simulink model "FOC1"  (R2022b)
settings: Solver=ode1  StartTime=0.0  StopTime=0.2  FixedStep=ctrlConst.TsSwitch  MaxStep=1e-6  RelTol=1e-3  EnableMultiTasking=on
undefined symbols (not defined in the file): ECM, f32_P_Coef, f32_P_Modulation, f32_P_SpdNeglimit_rpm, f32_P_SpdPoslimit_rpm, f32_P_SpeedPiMaxRatio, f32_P_SpeedPiMinRatio, FFW_enable, g_msgCore0to2_AcrKi, g_msgCore0to2_AcrKiStb, g_msgCore0to2_AcrKp, g_msgCore0to2_AcrKpStb, g_msgCore0to2_AcrSwtHiRpm, g_msgCore0to2_AcrSwtLoRpm, g_msgCore0to2_AfrKp, g_msgCore0to2_AfrTi, g_msgCore0to2_AsrKpHi, g_msgCore0to2_AsrKpLo, g_msgCore0to2_AsrSwtHiRpm, g_msgCore0to2_AsrSwtLoRpm, g_msgCore0to2_AsrTiHi, g_msgCore0to2_AsrTiLo, g_msgCore0to2_CalibEn, g_msgCore0to2_DecoupleEn, g_msgCore0to2_linearKpEn, g_msgCore0to2_maxCur, g_msgCore0to2_maxFwcCurRatio, g_msgCore0to2_maxTrq, g_msgCore0to2_pwmFrqSet, PWMFrqSwitch_C, SC_Ld_P, SC_Lq_P, SC_Psi_P, Spdratelimit_C, Tsw, u16_P_MotorPair
libraries: simulink x4, MathLib x2
(part 1 of 2)
settings Model: Creator=M00039784  LastModifiedBy=M00039784
settings SolverCC: AlgebraicLoopSolver=TrustRegion  InsertRTBMode=Never (minimum delay)
settings DataIOCC: LimitDataPoints=on  SaveFormat=Array  SaveOutput=off  SaveTime=off
settings OptimizationCC: DefaultParameterBehavior=Inlined  UseDivisionForNetSlopeComputation=on  UseFloatMulNetSlope=on  DefaultUnderspecifiedDataType=single  InlineInvariantSignals=on  PassReuseOutputArgsAs=Individual arguments  ExpressionDepthLimit=2147483647  ZeroExternalMemoryAtStartup=off  ZeroInternalMemoryAtStartup=off  NoFixptDivByZeroProtection=on  EfficientFloat2IntCast=on  LifeSpan=1  EfficientTunableParamExpr=on
settings DebuggingCC: ReadBeforeWriteMsg=DisableAll  WriteAfterWriteMsg=DisableAll  WriteAfterReadMsg=DisableAll  AlgebraicLoopMsg=none  MultiTaskDSMMsg=none  SingleTaskRateTransMsg=error  IntegerOverflowMsg=none  ParameterPrecisionLossMsg=none  FcnCallInpInsideContextMsg=warning  BusObjectLabelMismatch=none  AssertControl=DisableAll  AllowSymbolicDim=off  StateNameClashWarn=warning  SFUnexpectedBacktrackingDiag=warning  SFNoUnconditionalDefaultTransitionDiag=warning  SFExecutionAtInitializationDiag=none  SFMachineParentedDataDiag=warning  IntegerSaturationMsg=none  UnitsInconsistencyMsg=none  ArithmeticOperatorsInVariantConditions=warning
settings HardwareCC: ProdBitPerPointer=32  ProdBitPerSizeT=32  ProdBitPerPtrDiffT=32  ProdLargestAtomicFloat=None  ProdWordSize=32  ProdHWDeviceType=Infineon->TriCore
settings ModelReferenceCC: UpdateModelReferenceTargets=IfOutOfDate  EnableRefExpFcnMdlSchedulingChecks=on  ModelReferenceNumInstancesAllowed=Single  PropagateSignalLabelsOutOfModel=off
settings SFSimCC: SFSimEcho=off  SimUseLocalCustomCode=off  SimGenImportedTypeDefs=on  MATLABDynamicMemAlloc=off  CustomCodeUndefinedFunction=UseInterfaceOnly
settings RTWCC: Description=Embedded Coder  SystemTargetFile=ert.tlc  GenCodeOnly=on  GenerateMakefile=off  TemplateMakefile=ec_target.tmf  RTWVerbose=off  RTWUseLocalCustomCode=off  CodeExecutionProfiling=on  CodeProfilingSaveOptions=AllData  CodeProfilingInstrumentation=detailed
settings CodeAppCC: ForceParamTrailComments=on  IgnoreCustomStorageClasses=off  IgnoreTestpoints=on  MaxIdLength=64  SimulinkDataObjDesc=on  MATLABFcnDesc=on  CustomSymbolStrGlobalVar=pmsmfoc_rt$N$M  CustomSymbolStrType=pmsmfoc_$N$M  CustomSymbolStrFcn=$N$M$F  CustomSymbolStrFcnArg=$I$N$M  CustomSymbolStrMacro=$N$M  InsertBlockDesc=on  StateflowObjectComments=on  MATLABSourceComments=on  InternalIdentifier=Classic
settings ERTTargetCC: TargetLangStandard=C99 (ISO)  UtilityFuncGeneration=Shared location  MultiwordLength=2048  CombineSignalStateStructs=on  SupportAbsoluteTime=off  SupportNonFinite=off  SupportComplex=off  SupportNonInlinedSFcns=on  RemoveResetFunc=off  ParenthesesLevel=Maximum  GenerateASAP2=on  InlinedParameterPlacement=NonHierarchical  ERTCustomFileTemplate=example_file_process.tlc  EnableDataOwnership=on  ConvertIfToSwitch=off  SuppressUnreachableDefaultCases=off  MemSecPackage=Simulink  MemSecDataConstants=MemConst  MemSecDataParameters=MemConstVolatile
settings ConfigComp: CovMetricSettings=dcmtrzow  CovHTMLOptions=-aTS=1 -bRG=1 -bTC=1 -hTR=0 -nFC=0 -scm=1 -bcm=1 -xEv=0  CovSaveCumulativeToWorkspaceVar=on  CovSaveSingleToWorkspaceVar=on  CovExternalEMLEnable=off  CovSFcnEnable=off
settings SimscapeCC: SimscapeNormalizeSystem=off

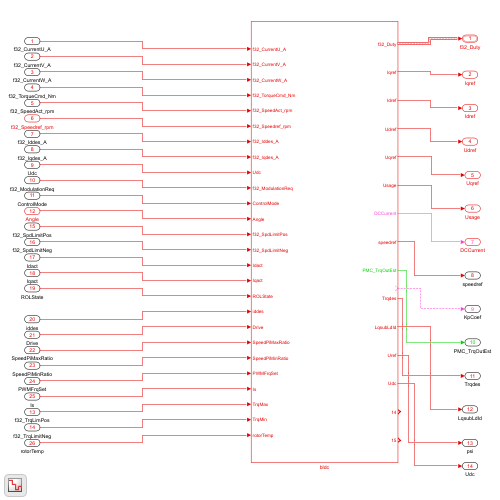
[thumbnail: Simulink's stored preview of the top-level diagram]
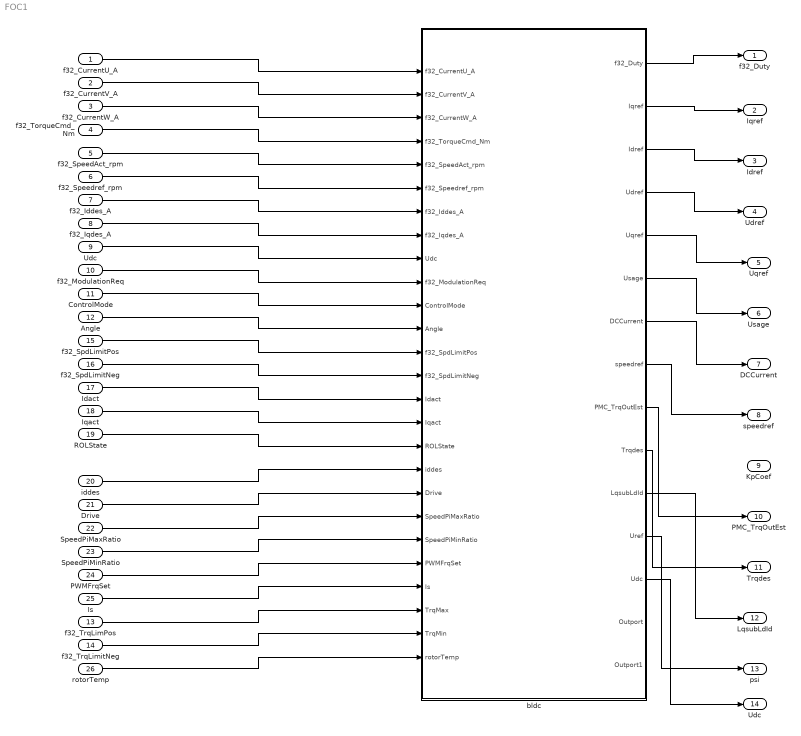
== system FOC1 ==
  f32_CurrentU_A : Inport  OutDataTypeStr=single  PortDimensions=1  SampleTime=0.0001
  f32_CurrentV_A : Inport  Port=2  OutDataTypeStr=single  PortDimensions=1  SampleTime=0.0001
  f32_CurrentW_A : Inport  Port=3  OutDataTypeStr=single  PortDimensions=1  SampleTime=0.0001
  f32_TorqueCmd_Nm : Inport  Port=4  OutDataTypeStr=single  PortDimensions=1
  f32_SpeedAct_rpm : Inport  Port=5  OutDataTypeStr=single  PortDimensions=1  SampleTime=0.0001
  f32_Speedref_rpm : Inport  Port=6  OutDataTypeStr=single  PortDimensions=1
  f32_Iddes_A : Inport  Port=7
  f32_Iqdes_A : Inport  Port=8
  "Udc " : Inport  Port=9  OutDataTypeStr=single  PortDimensions=1
  f32_ModulationReq : Inport  Port=10  OutDataTypeStr=single  PortDimensions=1
  ControlMode : Inport  Port=11  OutDataTypeStr=Enum: ECM  PortDimensions=1  SampleTime=0.0001
  Angle : Inport  Port=12  OutDataTypeStr=uint16  PortDimensions=1  SampleTime=0.0001
  f32_TrqLimPos : Inport  Port=13
  f32_TrqLimitNeg : Inport  Port=14
  f32_SpdLimitPos : Inport  Port=15
  f32_SpdLimitNeg : Inport  Port=16
  Idact : Inport  Port=17
  Iqact : Inport  Port=18
  ROLState : Inport  Port=19
  iddes : Inport  Port=20
  Drive : Inport  Port=21  OutDataTypeStr=boolean
  SpeedPiMaxRatio : Inport  Port=22  OutDataTypeStr=single
  SpeedPiMinRatio : Inport  Port=23  OutDataTypeStr=single
  PWMFrqSet : Inport  Port=24
  Is : Inport  Port=25
  rotorTemp : Inport  Port=26
  bldc : Subsystem
  f32_Duty : Outport  OutDataTypeStr=Bus: Duty
  Iqref : Outport  Port=2
  Idref : Outport  Port=3
  Udref : Outport  Port=4
  Uqref : Outport  Port=5
  Usage : Outport  Port=6
  DCCurrent : Outport  Port=7
  speedref : Outport  Port=8
  KpCoef : Outport  Port=9
  PMC_TrqOutEst : Outport  Port=10
  Trqdes : Outport  Port=11
  LqsubLdId : Outport  Port=12
  psi : Outport  Port=13
  Udc : Outport  Port=14
  wires:
  f32_SpdLimitPos/1 -> bldc/13(f32_SpdLimitPos)
  bldc/6(Usage) -> Usage/1
  f32_Speedref_rpm/1 -> bldc/6(f32_Speedref_rpm)
  f32_Iqdes_A/1 -> bldc/8(f32_Iqdes_A)
  bldc/2(Iqref) -> Iqref/1
  Angle/1 -> bldc/12(Angle)
  bldc/7(DCCurrent) -> DCCurrent/1
  bldc/5(Uqref) -> Uqref/1
  f32_SpdLimitNeg/1 -> bldc/14(f32_SpdLimitNeg)
  f32_CurrentU_A/1 -> bldc/1(f32_CurrentU_A)
  ControlMode/1 -> bldc/11(ControlMode)
  Iqact/1 -> bldc/16(Iqact)
  bldc/3(Idref) -> Idref/1
  f32_ModulationReq/1 -> bldc/10(f32_ModulationReq)
  f32_CurrentV_A/1 -> bldc/2(f32_CurrentV_A)
  bldc/1(f32_Duty) -> f32_Duty/1
  Idact/1 -> bldc/15(Idact)
  f32_TorqueCmd_Nm/1 -> bldc/4(f32_TorqueCmd_Nm)
  f32_SpeedAct_rpm/1 -> bldc/5(f32_SpeedAct_rpm)
  f32_Iddes_A/1 -> bldc/7(f32_Iddes_A)
  f32_CurrentW_A/1 -> bldc/3(f32_CurrentW_A)
  "Udc "/1 -> bldc/9("Udc ")
  bldc/4(Udref) -> Udref/1
  ROLState/1 -> bldc/17(ROLState)
  iddes/1 -> bldc/18(iddes)
  Drive/1 -> bldc/19(Drive)
  PWMFrqSet/1 -> bldc/22(PWMFrqSet)
  bldc/8(speedref) -> speedref/1
  Is/1 -> bldc/23(Is)
  ? -> KpCoef/1
  bldc/9(PMC_TrqOutEst) -> PMC_TrqOutEst/1
  f32_TrqLimPos/1 -> bldc/24(TrqMax)
  f32_TrqLimitNeg/1 -> bldc/25(TrqMin)
  SpeedPiMaxRatio/1 -> bldc/20(SpeedPiMaxRatio)
  SpeedPiMinRatio/1 -> bldc/21(SpeedPiMinRatio)
  rotorTemp/1 -> bldc/26(rotorTemp)
  bldc/10(Trqdes) -> Trqdes/1
  bldc/11(LqsubLdId) -> LqsubLdId/1
  bldc/12(Uref) -> psi/1
  bldc/13(Udc) -> Udc/1

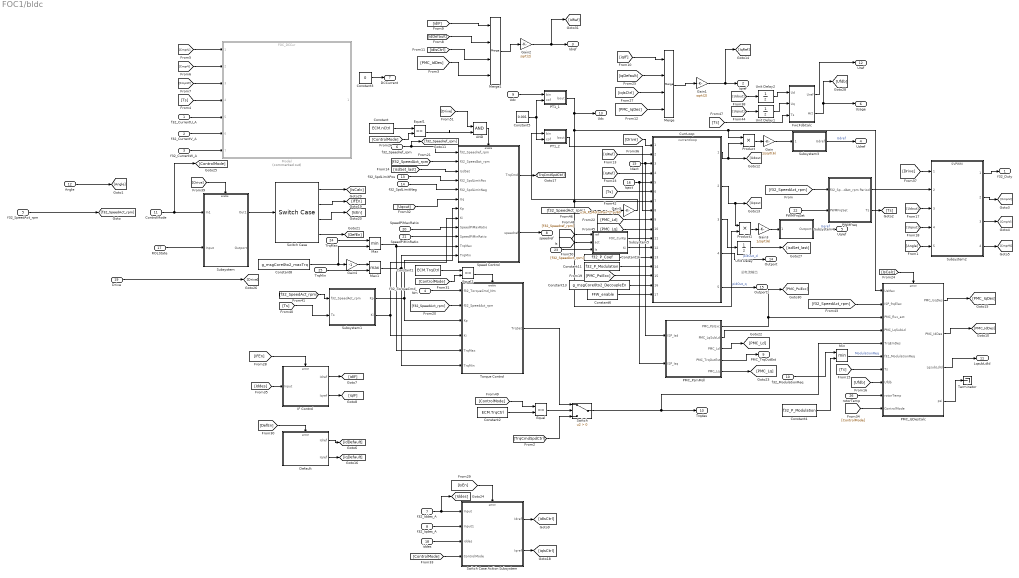
== system FOC1/bldc ==
  note: 总电流输出
  f32_CurrentU_A : Inport  OutDataTypeStr=single  PortDimensions=1  SampleTime=0.0001
  f32_CurrentV_A : Inport  Port=2  OutDataTypeStr=single  PortDimensions=1  SampleTime=0.0001
  f32_CurrentW_A : Inport  Port=3  OutDataTypeStr=single  PortDimensions=1  SampleTime=0.0001
  f32_TorqueCmd_Nm : Inport  Port=4  OutDataTypeStr=single  PortDimensions=1
  f32_SpeedAct_rpm : Inport  Port=5  OutDataTypeStr=single  PortDimensions=1  SampleTime=0.0001
  f32_Speedref_rpm : Inport  Port=6  OutDataTypeStr=single  PortDimensions=1  SampleTime=0.0001
  f32_Iddes_A : Inport  Port=7
  f32_Iqdes_A : Inport  Port=8
  "Udc " : Inport  Port=9  OutDataTypeStr=single  PortDimensions=1
  f32_ModulationReq : Inport  Port=10
  ControlMode : Inport  Port=11  OutDataTypeStr=Enum: ECM  PortDimensions=1  SampleTime=0.0001
  Angle : Inport  Port=12  OutDataTypeStr=uint16  PortDimensions=1  SampleTime=0.0001
  f32_SpdLimitPos : Inport  Port=13
  f32_SpdLimitNeg : Inport  Port=14
  Idact : Inport  Port=15
  Iqact : Inport  Port=16
  ROLState : Inport  Port=17
  iddes : Inport  Port=18
  Drive : Inport  Port=19
  SpeedPiMaxRatio : Inport  Port=20
  SpeedPiMinRatio : Inport  Port=21
  PWMFrqSet : Inport  Port=22
  Is : Inport  Port=23
  TrqMax : Inport  Port=24
  TrqMin : Inport  Port=25
  rotorTemp : Inport  Port=26
  AND : Logic  IconShape=distinctive  AllPortsSameDT=off  OutDataTypeStr=boolean
  Constant : Constant  Value=ECM.nCtrl
  Constant1 : Constant  Value=ECM.TrqCtrl
  Constant11 : Constant  Value=f32_P_Modulation
  Constant13 : Constant  Value=g_msgCore0to2_DecoupleEn
  Constant16 : Constant  Value=f32_P_Coef
  Constant2 : Constant  Value=ECM.TrqCtrl
  Constant3 : Constant  Value=0  OutDataTypeStr=single
  Constant4 : Constant  Value=f32_P_Modulation  OutDataTypeStr=single
  Constant5 : Constant  Value=0.001  OutDataTypeStr=single
  Constant6 : Constant  Value=FFW_enable
  Constant8 : Constant  Value=g_msgCore0to2_maxTrq  OutDataTypeStr=single  SampleTime=-1
  CurrLoop : ModelReference  ModelNameDialog=currentloop.slxp  ModelReferenceVersion=1.125  CopyOfModelProtected=on
  Default : Subsystem  TreatAsAtomicUnit=on
  Equal : RelationalOperator  Operator===  OutDataTypeStr=boolean  RndMeth=Simplest  InputSameDT=off
  Equal1 : RelationalOperator  Operator===  OutDataTypeStr=boolean  RndMeth=Simplest  InputSameDT=off
  Equal2 : RelationalOperator  Operator===  OutDataTypeStr=boolean  RndMeth=Simplest  InputSameDT=off
  FwcFdbCalc : Subsystem
  Gain : Gain  Gain=1/sqrt(6)
  Gain1 : Gain  Gain=sqrt(2)
  Gain2 : Gain  Gain=sqrt(2)
  Gain3 : Gain  Gain=1/sqrt(6)
  Gain4 : Gain  Gain=-1
  Gain5 : Gain  Gain=u16_P_MotorPair*2*pi/60
  IF Control : Subsystem  TreatAsAtomicUnit=on
  Max : MinMax  Inputs=2
  Max1 : MinMax  Function=max  Inputs=2
  Merge : Merge  Inputs=4  InitialOutput=0
  Merge1 : Merge  Inputs=4  InitialOutput=0
  Min : MinMax  Inputs=2
  Model : ModelReference  Commented=on  ModelNameDialog=FOC_DCCur.slx  SimulationMode=Normal  ModelReferenceVersion=1.20
  PMC_IsDesCalc : Subsystem
  PMC_PsmMdl : Subsystem
  PT1_1 : Subsystem
  PT1_2 : Subsystem
  PWMfreq : Subsystem
  Product : Product
  Product1 : Product
  Speed Control : Subsystem
  Subsystem : Subsystem
  Subsystem1 : Subsystem
  Subsystem2 : ModelReference  ModelNameDialog=SVPWM.slxp  ModelReferenceVersion=1.113  CopyOfModelProtected=on
  Subsystem3 : Subsystem
  Subsystem4 : Subsystem
  Subsystem5 : Subsystem
  Switch : Switch  Criteria=u2 > Threshold  SaturateOnIntegerOverflow=off  InputSameDT=off
  Switch Case : SwitchCase  CaseConditions={[ECM.nCtrl,ECM.TrqCtrl],ECM.IFCtrl,[ECM.IsCtrl,ECM.alOfsCal]}
  Switch Case Action Subsystem : Subsystem  TreatAsAtomicUnit=on
  Terminator : Terminator
  Torque Control : Subsystem
  Unit Delay : UnitDelay  SampleTime=-1  HasFrameUpgradeWarning=on
  Unit Delay1 : UnitDelay  SampleTime=-1  HasFrameUpgradeWarning=on
  Unit Delay2 : UnitDelay  SampleTime=-1  HasFrameUpgradeWarning=on
  f32_Duty : Outport  OutDataTypeStr=Bus: Duty
  Iqref : Outport  Port=2
  Idref : Outport  Port=3
  Udref : Outport  Port=4
  Uqref : Outport  Port=5
  Usage : Outport  Port=6
  DCCurrent : Outport  Port=7
  speedref : Outport  Port=8
  PMC_TrqOutEst : Outport  Port=9
  Trqdes : Outport  Port=10
  LqsubLdId : Outport  Port=11
  Uref : Outport  Port=12
  Udc : Outport  Port=13
  Outport : Outport  Port=14
  Outport1 : Outport  Port=15
  wires:
  Subsystem2/1 -> f32_Duty/1
  PWMfreq/1(Period) -> Subsystem2/2
  f32_CurrentW_A/1 -> Model/7
  CurrLoop/1 -> Product/2, [Udout]
  [Angle] -> Subsystem2/5
  f32_CurrentU_A/1 -> Model/5
  f32_SpeedAct_rpm/1 -> [f32_SpeedAct_rpm]
  f32_SpdLimitPos/1 -> Speed Control/4(f32_SpdLimitPos)
  f32_CurrentV_A/1 -> Model/6
  f32_SpdLimitNeg/1 -> Speed Control/5(f32_SpdLimitNeg)
  f32_Speedref_rpm/1 -> Speed Control/1(f32_Speedref_rpm), [f32_Speedref_rpm]
  CurrLoop/2 -> [Uqout], Product1/1
  PWMfreq/2(Ts) -> [Ts]
  [f32_SpeedAct_rpm] -> PWMfreq/1(f32_SpeedAct_rpm)
  ControlMode/1 -> [ControlMode], Subsystem/1(In1)
  Angle/1 -> [Angle]
  Idact/1 -> PMC_PsmMdl/1(ISP_Isd), CurrLoop/3
  Iqact/1 -> PMC_PsmMdl/2(ISP_Isq), CurrLoop/5
  [Ts] -> Model/4
  Subsystem2/2 -> [CmprU]
  Subsystem2/3 -> [CmprV]
  Subsystem2/4 -> [CmprW]
  [CmprW] -> Model/3
  [CmprV] -> Model/2
  [CmprU] -> Model/1
  Constant3/1 -> DCCurrent/1
  f32_Iddes_A/1 -> [Iddes], Switch Case Action Subsystem/1(Input)
  f32_Iqdes_A/1 -> Switch Case Action Subsystem/2(Input1)
  Default/1("Idref ") -> [idDefault]
  [idDefault] -> Merge1/2
  IF Control/1(Idref) -> [idIF]
  [idIF] -> Merge1/1
  IF Control/2(Iqref) -> [iqIF]
  Switch Case Action Subsystem/1("Idref ") -> [idIsCtrl]
  [idIsCtrl] -> Merge1/3
  [isdSet_last] -> Speed Control/3(IsdSet)
  [Udout] -> Subsystem2/3
  [Uqout] -> Subsystem2/4
  [f32_SpeedAct_rpm] -> Torque Control/2(f32_SpeedAct_rpm)
  [f32_SpeedAct_rpm] -> Speed Control/2(f32_SpeedAct_rpm)
  Merge/1 -> Gain1/1
  [IqRef] -> CurrLoop/4
  Default/2(Iqref) -> [iqDefault]
  Speed Control/1("TrqCmd ") -> [TrqCmdSpdCtrl]
  Switch Case Action Subsystem/2(Iqref) -> [iqIsCtrl]
  [IFEn] -> IF Control/Action
  Switch Case/2 -> [IFEn]
  [IsEn] -> Switch Case Action Subsystem/Action
  Switch Case/3 -> [IsEn]
  Switch Case/4 -> [DefEn]
  [DefEn] -> Default/Action
  Subsystem/1(Out1) -> Switch Case/1
  ROLState/1 -> Subsystem/2(Input)
  iddes/1 -> Switch Case Action Subsystem/3(iddes)
  [ControlMode] -> Switch Case Action Subsystem/4(ControlMode)
  [Iddes] -> IF Control/1(Input)
  Drive/1 -> [Drive]
  [Drive] -> CurrLoop/1
  [Drive] -> Subsystem2/1
  [Drive] -> Subsystem/Enable
  CurrLoop/3 -> Unit Delay/1
  Unit Delay/1 -> [isdSet_last]
  [Ts] -> Subsystem1/2(Ts)
  [f32_SpeedAct_rpm] -> Subsystem1/1(f32_SpeedAct_rpm)
  Subsystem1/1(Kp) -> Speed Control/7(Kp), Torque Control/3(Kp)
  Subsystem1/2(Ki) -> Speed Control/8(Ki), Torque Control/4(Ki)
  [Ts] -> CurrLoop/6
  PT1_1/1(bout) -> Udc/1, Product1/2, CurrLoop/7, Product/1, PMC_IsDesCalc/1(UsMax)
  SpeedPiMaxRatio/1 -> Speed Control/9(SpeedPiMaxRatio)
  SpeedPiMinRatio/1 -> Speed Control/10(SpeedPiMinRatio)
  PWMFrqSet/1 -> PWMfreq/2(PWMFrqSet)
  Speed Control/2(speedref) -> speedref/1
  Gain1/1 -> [IqRef], Iqref/1
  Product/1 -> Gain/1
  Product1/1 -> Gain3/1
  Subsystem4/1(Outport) -> Uqref/1  "Uqref"
  Gain/1 -> Subsystem3/1(" ")
  Subsystem3/1(Udref) -> Udref/1  "Udref"
  Gain3/1 -> Subsystem4/1(" ")
  PMC_PsmMdl/1(PMC_PsiExc) -> [PMC_PsiExc], PMC_IsDesCalc/3(PMC_flux_act)
  PMC_PsmMdl/2(PMC_LqSubLd) -> PMC_IsDesCalc/4(PMC_LqSubLd)
  PMC_PsmMdl/4(PMC_TrqOutEst) -> PMC_TrqOutEst/1
  Merge1/1 -> Gain2/1
  Gain2/1 -> [IdRef], Idref/1
  [IdRef] -> CurrLoop/2
  TrqMax/1 -> Max/1
  Constant8/1 -> Max/2, Gain4/1
  Gain4/1 -> Max1/1
  TrqMin/1 -> Max1/2
  Max/1 -> Torque Control/5(TrqMax), Speed Control/11(TrqMax)
  Max1/1 -> Speed Control/12(TrqMin), Torque Control/6(TrqMin)
  [ControlMode] -> Equal/1
  Constant2/1 -> Equal/2
  [TrqCmdSpdCtrl] -> Switch/3
  [f32_SpeedAct_rpm] -> PMC_IsDesCalc/2(ISP_frqElec)
  PMC_IsDesCalc/1(PMC_IsqDes) -> [PMC_IqDes]
  f32_TorqueCmd_Nm/1 -> Torque Control/1(f32_TorqueCmd_Nm)
  Torque Control/1(TrqSet) -> Switch/1
  Switch/1 -> Trqdes/1, PMC_IsDesCalc/5(TrqEmDes)
  [iqIF] -> Merge/1
  [iqDefault] -> Merge/2
  [iqIsCtrl] -> Merge/3
  [PMC_IdDes] -> Merge1/4
  [PMC_IqDes] -> Merge/4
  Equal/1 -> Switch/2
  Switch Case/1 -> [IsCalc]
  [IsCalc] -> PMC_IsDesCalc/Action
  Constant1/1 -> Equal2/1
  [ControlMode] -> Equal2/2
  Equal2/1 -> Torque Control/Enable
  PMC_IsDesCalc/2(PMC_IdDes) -> [PMC_IdDes]
  FwcFdbCalc/2(Act) -> [Ufdb], Usage/1
  [Ts] -> PMC_IsDesCalc/7(Ts)
  [Uqout] -> Speed Control/6(Uq)
  [Udout] -> Unit Delay2/1
  [Uqout] -> Unit Delay1/1
  rotorTemp/1 -> PMC_IsDesCalc/9(rotorTemp)
  PMC_PsmMdl/3(PMC_Ld) -> [PMC_Ld]
  PMC_PsmMdl/5(PMC_Lq) -> [PMC_Lq]
  PMC_IsDesCalc/3(LqsubLdId) -> LqsubLdId/1
  Unit Delay2/1 -> FwcFdbCalc/1(Ud)
  Unit Delay1/1 -> FwcFdbCalc/2(Uq)
  [Ts] -> FwcFdbCalc/3(Ts)
  Constant4/1 -> Min/2
  Min/1 -> PMC_IsDesCalc/6(f32_ModulationReq)  "ModulationReq"
  f32_ModulationReq/1 -> Min/1
  [Ufdb] -> PMC_IsDesCalc/8(Ufdb)
  PMC_IsDesCalc/4(psi) -> Terminator/1
  [f32_SpeedAct_rpm] -> Gain5/1
  [PMC_Ld] -> CurrLoop/9
  [PMC_Lq] -> CurrLoop/10
  Subsystem5/1(FOC_CurKp) -> CurrLoop/11
  Subsystem5/2(Ki) -> CurrLoop/12
  Constant16/1 -> CurrLoop/13
  [PMC_PsiExc] -> CurrLoop/15
  Constant11/1 -> CurrLoop/14
  Constant13/1 -> CurrLoop/16
  Constant6/1 -> CurrLoop/17
  Gain5/1 -> PT1_2/1(bin)
  AND/1 -> Speed Control/Enable
  Equal1/1 -> AND/2
  Constant/1 -> Equal1/1
  [ControlMode] -> Equal1/2
  [Drive] -> AND/1
  Is/1 -> Subsystem5/3(Is)
  [f32_Speedref_rpm] -> Subsystem5/1(ref)
  [f32_SpeedAct_rpm] -> Subsystem5/2(act)
  "Udc "/1 -> PT1_1/1(bin)
  Constant5/1 -> PT1_2/2(cof), PT1_1/2(cof)
  PT1_2/1(bout) -> CurrLoop/8
  [ControlMode] -> PMC_IsDesCalc/10(ControlMode)
  FwcFdbCalc/1(Uref) -> Uref/1
  CurrLoop/5 -> Outport1/1  "pidOut_q"
  CurrLoop/4 -> Outport/1  "pidOut_d"

== system FOC1/bldc/Default ==
  Action Port : ActionPort  InitializeStates=reset  ActionPortLabel=default:
  Constant : Constant  Value=0  OutDataTypeStr=single
  Constant1 : Constant  Value=0  OutDataTypeStr=single
  "Idref " : Outport  VectorParamsAs1DForOutWhenUnconnected=off
  Iqref : Outport  Port=2  VectorParamsAs1DForOutWhenUnconnected=off
  wires:
  Constant1/1 -> Iqref/1
  Constant/1 -> "Idref "/1

== system FOC1/bldc/FwcFdbCalc ==
  Ud : Inport
  Uq : Inport  Port=2
  Ts : Inport  Port=3
  Add : Sum
  Constant1 : Constant  Value=500  OutDataTypeStr=single
  PT1_1 : Subsystem
  Product : Product  OutDataTypeStr=single
  Product1 : Product  OutDataTypeStr=single
  Product2 : Product
  Sqrt : Sqrt
  Uref : Outport
  Act : Outport  Port=2  VectorParamsAs1DForOutWhenUnconnected=off
  wires:
  Uq/1 -> Product1/2, Product1/1
  Add/1 -> Sqrt/1
  Product1/1 -> Add/2
  Ud/1 -> Product/2, Product/1
  Product/1 -> Add/1
  Sqrt/1 -> Uref/1, PT1_1/1(bin)
  PT1_1/1(bout) -> Act/1
  Product2/1 -> PT1_1/2(cof)
  Constant1/1 -> Product2/2
  Ts/1 -> Product2/1

== system FOC1/bldc/IF Control ==
  Input : Inport
  Action Port : ActionPort  InitializeStates=reset  ActionPortLabel=case [ IFCtrl ]:
  Constant1 : Constant  Value=0  OutDataTypeStr=single
  Idref : Outport  InitialOutput=0  VectorParamsAs1DForOutWhenUnconnected=off
  Iqref : Outport  Port=2  InitialOutput=0
  wires:
  Input/1 -> Idref/1
  Constant1/1 -> Iqref/1

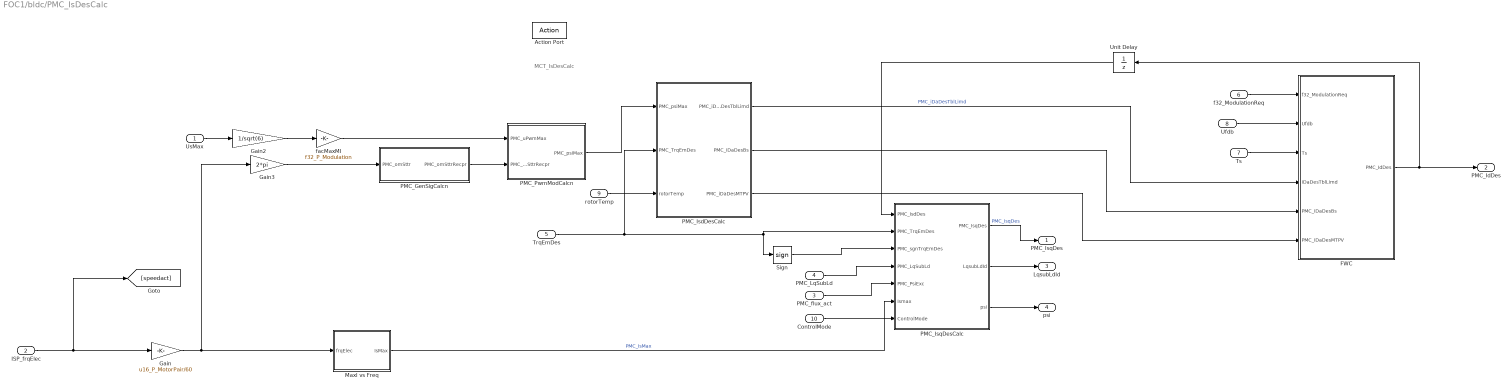
== system FOC1/bldc/PMC_IsDesCalc ==
  note: MCT_IsDesCalc
  UsMax : Inport
  ISP_frqElec : Inport  Port=2
  PMC_flux_act : Inport  Port=3
  PMC_LqSubLd : Inport  Port=4
  TrqEmDes : Inport  Port=5
  f32_ModulationReq : Inport  Port=6  OutDataTypeStr=single  PortDimensions=1
  Ts : Inport  Port=7
  Ufdb : Inport  Port=8
  rotorTemp : Inport  Port=9
  ControlMode : Inport  Port=10
  Action Port : ActionPort  InitializeStates=reset  ActionPortLabel=case [ nCtrl TrqCtrl ]:
  FWC : Subsystem
  Gain : Gain  Gain=u16_P_MotorPair/60
  Gain2 : Gain  Gain=1/sqrt(6)
  Gain3 : Gain  Gain=2*pi
  MaxI vs Freq : Subsystem
  PMC_GenSigCalcn : Subsystem  TreatAsAtomicUnit=on  SystemSampleTime=Tsw
  PMC_IsdDesCalc : Subsystem  TreatAsAtomicUnit=on  SystemSampleTime=Tsw
  PMC_IsqDesCalc : Subsystem  TreatAsAtomicUnit=on  SystemSampleTime=Tsw
  PMC_PwmModCalcn : Subsystem  TreatAsAtomicUnit=on  SystemSampleTime=Tsw
  Sign : Signum
  Unit Delay : UnitDelay  SampleTime=-1  HasFrameUpgradeWarning=on
  facMaxMI : Gain  Gain=f32_P_Modulation  ParamDataTypeStr=single
  PMC_IsqDes : Outport  InitialOutput=0  VectorParamsAs1DForOutWhenUnconnected=off
  PMC_IdDes : Outport  Port=2  InitialOutput=0
  LqsubLdId : Outport  Port=3
  psi : Outport  Port=4
  wires:
  Gain3/1 -> PMC_GenSigCalcn/1(PMC_omSttr)
  PMC_GenSigCalcn/1(PMC_omSttrRecpr) -> PMC_PwmModCalcn/2(PMC_omSttrRecpr)
  facMaxMI/1 -> PMC_PwmModCalcn/1(PMC_uPwmMax)
  PMC_LqSubLd/1 -> PMC_IsqDesCalc/4(PMC_LqSubLd)
  PMC_flux_act/1 -> PMC_IsqDesCalc/5(PMC_PsiExc)
  Sign/1 -> PMC_IsqDesCalc/3(PMC_sgnTrqEmDes)
  TrqEmDes/1 -> PMC_IsdDesCalc/2(PMC_TrqEmDes), Sign/1, PMC_IsqDesCalc/2(PMC_TrqEmDes)
  PMC_PwmModCalcn/1(PMC_psiMax) -> PMC_IsdDesCalc/1(PMC_psiMax)
  Gain/1 -> Gain3/1, MaxI vs Freq/1(frqElec)
  UsMax/1 -> Gain2/1
  ISP_frqElec/1 -> [speedact], Gain/1
  PMC_IsqDesCalc/1(PMC_IsqDes) -> PMC_IsqDes/1  "PMC_IsqDes"
  MaxI vs Freq/1(IsMax) -> PMC_IsqDesCalc/6(Ismax)  "PMC_IsMax"
  PMC_IsdDesCalc/1(PMC_iDaDesTblLimd) -> FWC/4(iDaDesTblLimd)  "PMC_iDaDesTblLimd"
  FWC/1(PMC_IdDes) -> Unit Delay/1, PMC_IdDes/1
  Gain2/1 -> facMaxMI/1
  f32_ModulationReq/1 -> FWC/1(f32_ModulationReq)
  Ufdb/1 -> FWC/2(Ufdb)
  PMC_IsdDesCalc/3(PMC_iDaDesMTPV) -> FWC/6(PMC_iDaDesMTPV)
  Ts/1 -> FWC/3(Ts)
  PMC_IsdDesCalc/2(PMC_iDaDesBs) -> FWC/5(PMC_iDaDesBs)
  Unit Delay/1 -> PMC_IsqDesCalc/1(PMC_IsdDes)
  rotorTemp/1 -> PMC_IsdDesCalc/3(rotorTemp)
  PMC_IsqDesCalc/2(LqsubLdId) -> LqsubLdId/1
  PMC_IsqDesCalc/3(psi) -> psi/1
  ControlMode/1 -> PMC_IsqDesCalc/7(ControlMode)

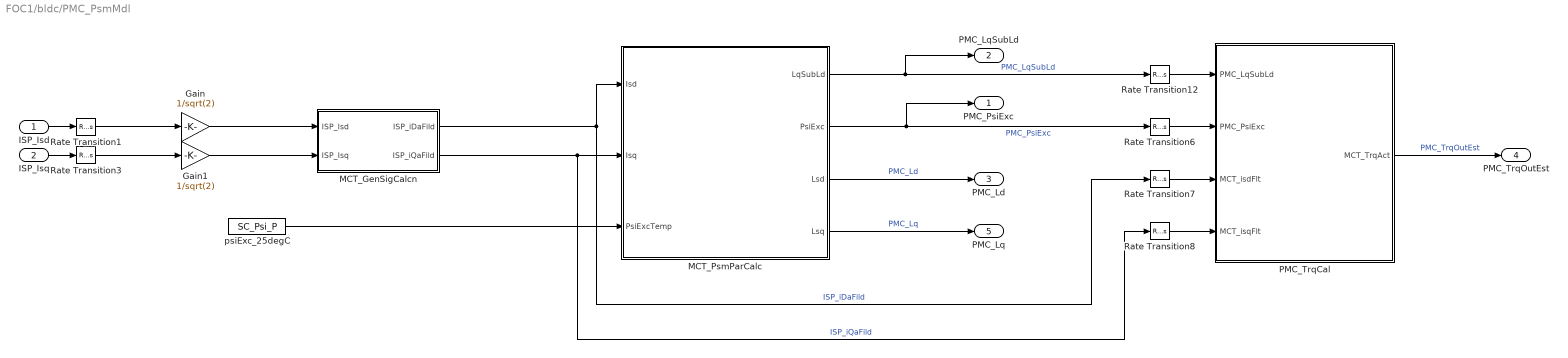
== system FOC1/bldc/PMC_PsmMdl ==
  ISP_Isd : Inport
  ISP_Isq : Inport  Port=2
  Gain : Gain  Gain=1/sqrt(2)
  Gain1 : Gain  Gain=1/sqrt(2)
  MCT_GenSigCalcn : Subsystem
  MCT_PsmParCalc : Subsystem  TreatAsAtomicUnit=on
  PMC_TrqCal : Subsystem
  Rate Transition1 : RateTransition  OutPortSampleTime=Tsw
  Rate Transition{6..8,12} (4 alike) : RateTransition  OutPortSampleTime=Ts_10ms
  Rate Transition3 : RateTransition  OutPortSampleTime=Tsw
  psiExc_25degC : Constant  Value=SC_Psi_P  OutDataTypeStr=single  SampleTime=-1
  PMC_PsiExc : Outport  VectorParamsAs1DForOutWhenUnconnected=off
  PMC_LqSubLd : Outport  Port=2  VectorParamsAs1DForOutWhenUnconnected=off
  PMC_Ld : Outport  Port=3  VectorParamsAs1DForOutWhenUnconnected=off
  PMC_TrqOutEst : Outport  Port=4
  PMC_Lq : Outport  Port=5
  wires:
  MCT_PsmParCalc/1(LqSubLd) -> Rate Transition12/1, PMC_LqSubLd/1  "PMC_LqSubLd"
  MCT_PsmParCalc/2(PsiExc) -> PMC_PsiExc/1, Rate Transition6/1  "PMC_PsiExc"
  Rate Transition3/1 -> Gain1/1
  Rate Transition1/1 -> Gain/1
  MCT_GenSigCalcn/1(ISP_iDaFild) -> MCT_PsmParCalc/1(Isd), Rate Transition7/1  "ISP_iDaFild"
  ISP_Isq/1 -> Rate Transition3/1
  ISP_Isd/1 -> Rate Transition1/1
  MCT_GenSigCalcn/2(ISP_iQaFild) -> Rate Transition8/1, MCT_PsmParCalc/2(Isq)  "ISP_iQaFild"
  MCT_PsmParCalc/3(Lsd) -> PMC_Ld/1  "PMC_Ld"
  MCT_PsmParCalc/4(Lsq) -> PMC_Lq/1  "PMC_Lq"
  psiExc_25degC/1 -> MCT_PsmParCalc/3(PsiExcTemp)
  Rate Transition12/1 -> PMC_TrqCal/1(PMC_LqSubLd)
  Rate Transition6/1 -> PMC_TrqCal/2(PMC_PsiExc)
  Rate Transition7/1 -> PMC_TrqCal/3(MCT_isdFlt)
  Rate Transition8/1 -> PMC_TrqCal/4(MCT_isqFlt)
  PMC_TrqCal/1(MCT_TrqAct) -> PMC_TrqOutEst/1  "PMC_TrqOutEst"
  Gain/1 -> MCT_GenSigCalcn/1(ISP_Isd)
  Gain1/1 -> MCT_GenSigCalcn/2(ISP_Isq)

== system FOC1/bldc/PT1_1 ==
  bin : Inport
  cof : Inport  Port=2
  Constant : Constant  OutDataTypeStr=single
  Product1 : Product  RndMeth=Zero  OutDataTypeStr=Inherit: Same as first input
  Product3 : Product  RndMeth=Zero  OutDataTypeStr=Inherit: Same as first input
  Subtract : Sum  Inputs=-+  OutDataTypeStr=Inherit: Same as first input
  Sum1 : Sum  Inputs=|++  OutDataTypeStr=Inherit: Same as first input
  Unit Delay1 : UnitDelay  SampleTime=-1  HasFrameUpgradeWarning=on
  bout : Outport  VectorParamsAs1DForOutWhenUnconnected=off
  wires:
  Product3/1 -> Sum1/2
  Unit Delay1/1 -> Product3/1
  Product1/1 -> Sum1/1
  bin/1 -> Product1/1
  Constant/1 -> Subtract/2
  cof/1 -> Subtract/1, Product1/2
  Sum1/1 -> bout/1, Unit Delay1/1
  Subtract/1 -> Product3/2

== system FOC1/bldc/PT1_2 ==
  bin : Inport
  cof : Inport  Port=2
  Constant : Constant  OutDataTypeStr=single
  Product1 : Product  RndMeth=Zero  OutDataTypeStr=Inherit: Same as first input
  Product3 : Product  RndMeth=Zero  OutDataTypeStr=Inherit: Same as first input
  Subtract : Sum  Inputs=-+  OutDataTypeStr=Inherit: Same as first input
  Sum1 : Sum  Inputs=|++  OutDataTypeStr=Inherit: Same as first input
  Unit Delay1 : UnitDelay  SampleTime=-1  HasFrameUpgradeWarning=on
  bout : Outport  VectorParamsAs1DForOutWhenUnconnected=off
  wires:
  Subtract/1 -> Product3/2
  Sum1/1 -> Unit Delay1/1, bout/1
  cof/1 -> Product1/2, Subtract/1
  Constant/1 -> Subtract/2
  bin/1 -> Product1/1
  Product1/1 -> Sum1/1
  Unit Delay1/1 -> Product3/1
  Product3/1 -> Sum1/2

== system FOC1/bldc/PWMfreq ==
  f32_SpeedAct_rpm : Inport
  PWMFrqSet : Inport  Port=2
  1-D Lookup Table : Lookup_n-D  Commented=on  NumberOfTableDimensions=1  BreakpointsForDimension1=[0 400 800]  Table=[5000;5000;5000]  InternalRulePriority=Speed  OutDataTypeStr=uint32  RndMeth=Simplest
  Constant : Constant  Value=g_msgCore0to2_pwmFrqSet  OutDataTypeStr=single
  Constant1 : Constant  OutDataTypeStr=single
  Constant2 : Constant  Value=PWMFrqSwitch_C
  Divide : Product  Inputs=*/
  Gain : Gain  Gain=100000000  OutDataTypeStr=uint32
  Switch : Switch  Criteria=u2 > Threshold  SaturateOnIntegerOverflow=off  InputSameDT=off
  Period : Outport  OutDataTypeStr=uint32  VectorParamsAs1DForOutWhenUnconnected=off
  Ts : Outport  Port=2  OutDataTypeStr=single
  wires:
  Constant/1 -> Switch/3
  f32_SpeedAct_rpm/1 -> 1-D Lookup Table/1
  Divide/1 -> Gain/1, Ts/1
  Constant1/1 -> Divide/1
  Gain/1 -> Period/1
  PWMFrqSet/1 -> Switch/1
  Switch/1 -> Divide/2
  Constant2/1 -> Switch/2

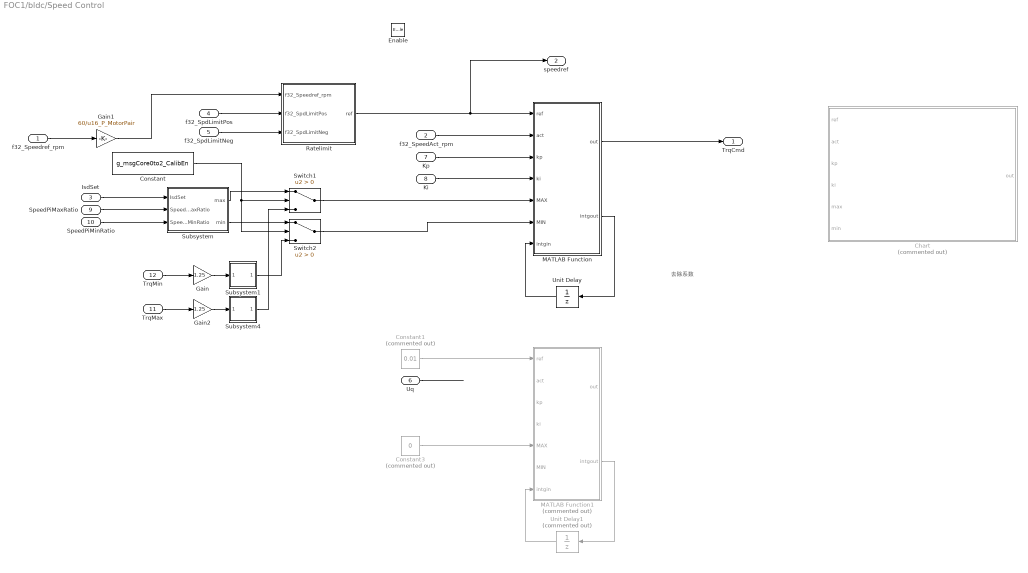
== system FOC1/bldc/Speed Control ==
  note: 去除系数
  f32_Speedref_rpm : Inport
  f32_SpeedAct_rpm : Inport  Port=2
  IsdSet : Inport  Port=3
  f32_SpdLimitPos : Inport  Port=4
  f32_SpdLimitNeg : Inport  Port=5
  Uq : Inport  Port=6
  Kp : Inport  Port=7
  Ki : Inport  Port=8
  SpeedPiMaxRatio : Inport  Port=9
  SpeedPiMinRatio : Inport  Port=10
  TrqMax : Inport  Port=11
  TrqMin : Inport  Port=12
  Enable : EnablePort  StatesWhenEnabling=reset
  Chart : Stateflow chart  Commented=on  TreatAsAtomicUnit=on
  Constant : Constant  Value=g_msgCore0to2_CalibEn
  Constant1 : Constant  Commented=on  Value=0.01
  Constant3 : Constant  Commented=on  Value=0
  Gain : Gain  Gain=1.25
  Gain1 : Gain  Gain=60/u16_P_MotorPair
  Gain2 : Gain  Gain=1.25
  MATLAB Function : MATLAB Function  TreatAsAtomicUnit=on
  MATLAB Function1 : MATLAB Function  Commented=on  TreatAsAtomicUnit=on
  Ratelimit : Subsystem
  Subsystem : Subsystem
  Subsystem1 : Subsystem
  Subsystem4 : Subsystem
  Switch1 : Switch  Criteria=u2 > Threshold  SaturateOnIntegerOverflow=off  InputSameDT=off
  Switch2 : Switch  Criteria=u2 > Threshold  SaturateOnIntegerOverflow=off  InputSameDT=off
  Unit Delay : UnitDelay  SampleTime=-1  HasFrameUpgradeWarning=on
  Unit Delay1 : UnitDelay  Commented=on  SampleTime=-1  HasFrameUpgradeWarning=on
  "TrqCmd " : Outport  OutputWhenDisabled=reset  InitialOutput=0
  speedref : Outport  Port=2  OutputWhenDisabled=reset  InitialOutput=0
  wires:
  Gain1/1 -> Ratelimit/1(f32_Speedref_rpm)
  IsdSet/1 -> Subsystem/1(IsdSet)
  Switch2/1 -> MATLAB Function/6(MIN)
  Switch1/1 -> MATLAB Function/5(MAX)
  f32_SpeedAct_rpm/1 -> MATLAB Function/2(act)
  Ratelimit/1(ref) -> speedref/1, MATLAB Function/1(ref)
  f32_SpdLimitPos/1 -> Ratelimit/2(f32_SpdLimitPos)
  f32_SpdLimitNeg/1 -> Ratelimit/3(f32_SpdLimitNeg)
  MATLAB Function/1(out) -> "TrqCmd "/1
  MATLAB Function/2(intgout) -> Unit Delay/1
  Unit Delay/1 -> MATLAB Function/7(intgin)
  f32_Speedref_rpm/1 -> Gain1/1
  Kp/1 -> MATLAB Function/3(kp)
  Ki/1 -> MATLAB Function/4(ki)
  SpeedPiMaxRatio/1 -> Subsystem/2(SpeedPiMaxRatio)
  SpeedPiMinRatio/1 -> Subsystem/3(SpeedPiMinRatio)
  Subsystem/1(max) -> Switch1/1
  Subsystem/2(min) -> Switch2/1
  TrqMax/1 -> Gain2/1
  TrqMin/1 -> Gain/1
  Constant/1 -> Switch1/2, Switch2/2
  Uq/1 -> ?
  Constant1/1 -> MATLAB Function1/1(ref)
  Constant3/1 -> MATLAB Function1/5(MAX)
  MATLAB Function1/2(intgout) -> Unit Delay1/1
  Unit Delay1/1 -> MATLAB Function1/7(intgin)
  Gain/1 -> Subsystem1/1(" ")
  Gain2/1 -> Subsystem4/1(" ")
  Subsystem4/1(Outport) -> Switch1/3
  Subsystem1/1(Outport) -> Switch2/3

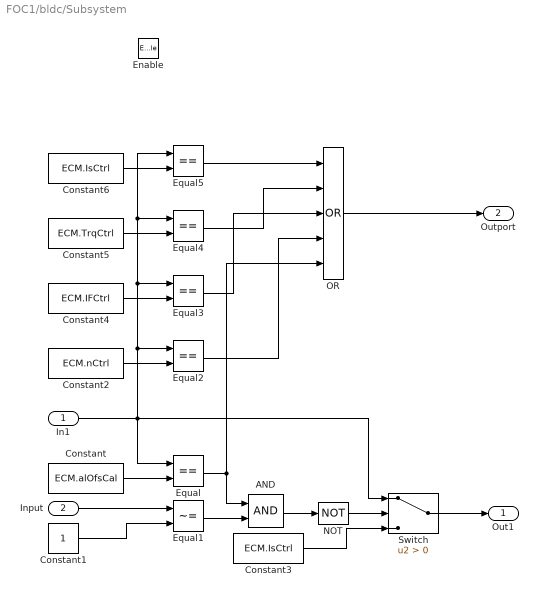
== system FOC1/bldc/Subsystem ==
  In1 : Inport
  Input : Inport  Port=2
  Enable : EnablePort  StatesWhenEnabling=reset
  AND : Logic  AllPortsSameDT=off  OutDataTypeStr=boolean
  Constant : Constant  Value=ECM.alOfsCal
  Constant1 : Constant  OutDataTypeStr=uint8
  Constant2 : Constant  Value=ECM.nCtrl
  Constant3 : Constant  Value=ECM.IsCtrl
  Constant4 : Constant  Value=ECM.IFCtrl
  Constant5 : Constant  Value=ECM.TrqCtrl
  Constant6 : Constant  Value=ECM.IsCtrl
  Equal{,2..5} (5 alike) : RelationalOperator  Operator===  OutDataTypeStr=boolean  RndMeth=Simplest  InputSameDT=off
  Equal1 : RelationalOperator  Operator=~=  OutDataTypeStr=boolean  RndMeth=Simplest  InputSameDT=off
  NOT : Logic  Operator=NOT  IconShape=distinctive  AllPortsSameDT=off  OutDataTypeStr=boolean
  OR : Logic  Operator=OR  Inputs=5  AllPortsSameDT=off  OutDataTypeStr=boolean
  Switch : Switch  Criteria=u2 > Threshold  SaturateOnIntegerOverflow=off  InputSameDT=off
  Out1 : Outport  OutputWhenDisabled=reset  InitialOutput=ECM.Init
  Outport : Outport  Port=2  OutputWhenDisabled=reset  InitialOutput=0
  wires:
  Constant/1 -> Equal/2
  Equal/1 -> OR/5, AND/1
  Input/1 -> Equal1/1
  Equal1/1 -> AND/2
  Constant1/1 -> Equal1/2
  AND/1 -> NOT/1
  NOT/1 -> Switch/2
  Switch/1 -> Out1/1
  Constant3/1 -> Switch/3
  Constant2/1 -> Equal2/2
  Constant4/1 -> Equal3/2
  Constant5/1 -> Equal4/2
  Constant6/1 -> Equal5/2
  In1/1 -> Equal5/1, Equal4/1, Equal3/1, Equal2/1, Equal/1, Switch/1
  Equal5/1 -> OR/1
  Equal4/1 -> OR/2
  Equal3/1 -> OR/3
  Equal2/1 -> OR/4
  OR/1 -> Outport/1

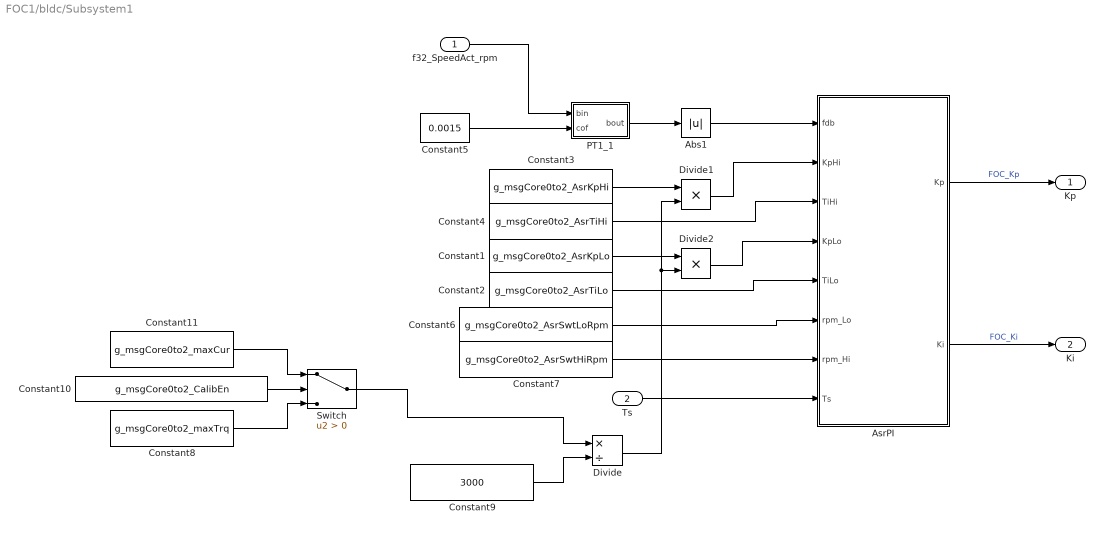
== system FOC1/bldc/Subsystem1 ==
  f32_SpeedAct_rpm : Inport
  Ts : Inport  Port=2
  Abs1 : Abs  SaturateOnIntegerOverflow=off
  AsrPI : MATLAB Function
  Constant1 : Constant  Value=g_msgCore0to2_AsrKpLo
  Constant10 : Constant  Value=g_msgCore0to2_CalibEn
  Constant11 : Constant  Value=g_msgCore0to2_maxCur  OutDataTypeStr=single  SampleTime=-1
  Constant2 : Constant  Value=g_msgCore0to2_AsrTiLo
  Constant3 : Constant  Value=g_msgCore0to2_AsrKpHi
  Constant4 : Constant  Value=g_msgCore0to2_AsrTiHi
  Constant5 : Constant  Value=0.0015  OutDataTypeStr=single
  Constant6 : Constant  Value=g_msgCore0to2_AsrSwtLoRpm
  Constant7 : Constant  Value=g_msgCore0to2_AsrSwtHiRpm
  Constant8 : Constant  Value=g_msgCore0to2_maxTrq  OutDataTypeStr=single  SampleTime=-1
  Constant9 : Constant  Value=3000  OutDataTypeStr=single  SampleTime=-1
  Divide : Product  Inputs=*/  OutDataTypeStr=single
  Divide1 : Product  Inputs=**  OutDataTypeStr=single
  Divide2 : Product  Inputs=**  OutDataTypeStr=single
  PT1_1 : Subsystem
  Switch : Switch  Criteria=u2 > Threshold  SaturateOnIntegerOverflow=off  InputSameDT=off
  Kp : Outport
  Ki : Outport  Port=2
  wires:
  f32_SpeedAct_rpm/1 -> PT1_1/1(bin)
  Constant5/1 -> PT1_1/2(cof)
  PT1_1/1(bout) -> Abs1/1
  Abs1/1 -> AsrPI/1(fdb)
  Constant4/1 -> AsrPI/3(TiHi)
  Constant2/1 -> AsrPI/5(TiLo)
  Constant6/1 -> AsrPI/6(rpm_Lo)
  Constant7/1 -> AsrPI/7(rpm_Hi)
  Ts/1 -> AsrPI/8(Ts)
  Constant9/1 -> Divide/2
  Constant3/1 -> Divide1/1
  Divide/1 -> Divide2/2, Divide1/2
  Divide1/1 -> AsrPI/2(KpHi)
  Constant1/1 -> Divide2/1
  Divide2/1 -> AsrPI/4(KpLo)
  Constant10/1 -> Switch/2
  Constant11/1 -> Switch/1
  Switch/1 -> Divide/1
  Constant8/1 -> Switch/3
  AsrPI/1(Kp) -> Kp/1  "FOC_Kp"
  AsrPI/2(Ki) -> Ki/1  "FOC_Ki"

== system FOC1/bldc/Subsystem3 ==
  " " : Inport
  Constant : Constant  Value=0.1  OutDataTypeStr=single
  Constant1 : Constant  OutDataTypeStr=single
  Minus : Sum  Inputs=+-
  Plus : Sum
  Product : Product
  Product1 : Product
  Unit Delay : UnitDelay  SampleTime=-1  HasFrameUpgradeWarning=on
  Udref : Outport
  wires:
  Plus/1 -> Udref/1, Unit Delay/1
  " "/1 -> Product/2
  Constant/1 -> Minus/2, Product/1
  Minus/1 -> Product1/2
  Product1/1 -> Plus/1
  Constant1/1 -> Minus/1
  Unit Delay/1 -> Product1/1
  Product/1 -> Plus/2

== system FOC1/bldc/Subsystem4 ==
  " " : Inport
  Constant : Constant  Value=0.1  OutDataTypeStr=single
  Constant1 : Constant  OutDataTypeStr=single
  Minus : Sum  Inputs=+-
  Plus : Sum
  Product : Product
  Product1 : Product
  Unit Delay : UnitDelay  SampleTime=-1  HasFrameUpgradeWarning=on
  Outport : Outport
  wires:
  Plus/1 -> Outport/1, Unit Delay/1
  " "/1 -> Product/2
  Constant/1 -> Minus/2, Product/1
  Minus/1 -> Product1/2
  Product1/1 -> Plus/1
  Constant1/1 -> Minus/1
  Unit Delay/1 -> Product1/1
  Product/1 -> Plus/2

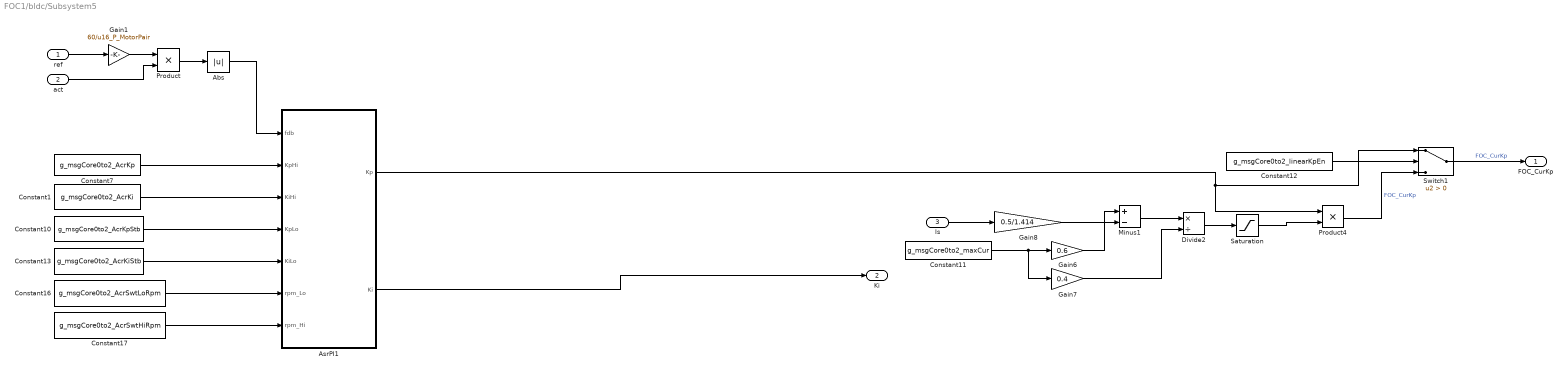
== system FOC1/bldc/Subsystem5 ==
  ref : Inport
  act : Inport  Port=2
  Is : Inport  Port=3
  Abs : Abs  SaturateOnIntegerOverflow=off
  AsrPI1 : MATLAB Function
  Constant1 : Constant  Value=g_msgCore0to2_AcrKi
  Constant10 : Constant  Value=g_msgCore0to2_AcrKpStb
  Constant11 : Constant  Value=g_msgCore0to2_maxCur
  Constant12 : Constant  Value=g_msgCore0to2_linearKpEn
  Constant13 : Constant  Value=g_msgCore0to2_AcrKiStb
  Constant16 : Constant  Value=g_msgCore0to2_AcrSwtLoRpm
  Constant17 : Constant  Value=g_msgCore0to2_AcrSwtHiRpm
  Constant7 : Constant  Value=g_msgCore0to2_AcrKp
  Divide2 : Product  Inputs=*/
  Gain1 : Gain  Gain=60/u16_P_MotorPair
  Gain6 : Gain  Gain=0.6
  Gain7 : Gain  Gain=0.4
  Gain8 : Gain  Gain=0.5/1.414
  Minus1 : Sum  Inputs=+-
  Product : Product
  Product4 : Product
  Saturation : Saturate  UpperLimit=1  LowerLimit=0.5
  Switch1 : Switch  Criteria=u2 > Threshold  SaturateOnIntegerOverflow=off  InputSameDT=off
  FOC_CurKp : Outport
  Ki : Outport  Port=2
  wires:
  Gain8/1 -> Minus1/2
  Constant11/1 -> Gain7/1, Gain6/1
  Constant16/1 -> AsrPI1/6(rpm_Lo)
  AsrPI1/1(Kp) -> Switch1/1, Product4/1
  Constant7/1 -> AsrPI1/2(KpHi)
  Minus1/1 -> Divide2/1
  Constant10/1 -> AsrPI1/4(KpLo)
  Constant13/1 -> AsrPI1/5(KiLo)
  Constant17/1 -> AsrPI1/7(rpm_Hi)
  Gain7/1 -> Divide2/2
  Constant12/1 -> Switch1/2
  Constant1/1 -> AsrPI1/3(KiHi)
  Divide2/1 -> Saturation/1
  Saturation/1 -> Product4/2
  Switch1/1 -> FOC_CurKp/1  "FOC_CurKp"
  Gain6/1 -> Minus1/1
  Product4/1 -> Switch1/3  "FOC_CurKp"
  AsrPI1/2(Ki) -> Ki/1
  Is/1 -> Gain8/1
  ref/1 -> Gain1/1
  Gain1/1 -> Product/1
  act/1 -> Product/2
  Product/1 -> Abs/1
  Abs/1 -> AsrPI1/1(fdb)

== system FOC1/bldc/Switch Case Action Subsystem ==
  Input : Inport
  Input1 : Inport  Port=2
  iddes : Inport  Port=3
  ControlMode : Inport  Port=4
  Action Port : ActionPort  ActionPortLabel=case [ IsCtrl alOfsCal ]:
  Constant : Constant  Value=ECM.alOfsCal
  Constant1 : Constant  Value=0  OutDataTypeStr=single
  Equal : RelationalOperator  Operator===  OutDataTypeStr=boolean  RndMeth=Simplest  InputSameDT=off
  Switch : Switch  Criteria=u2 > Threshold  SaturateOnIntegerOverflow=off  InputSameDT=off
  Switch1 : Switch  Criteria=u2 > Threshold  SaturateOnIntegerOverflow=off  InputSameDT=off
  "Idref " : Outport  InitialOutput=0  VectorParamsAs1DForOutWhenUnconnected=off
  Iqref : Outport  Port=2  InitialOutput=0  VectorParamsAs1DForOutWhenUnconnected=off
  wires:
  ControlMode/1 -> Equal/1
  Constant/1 -> Equal/2
  Switch/1 -> "Idref "/1
  Switch1/1 -> Iqref/1
  Equal/1 -> Switch1/2, Switch/2
  Input/1 -> Switch/3
  Input1/1 -> Switch1/3
  iddes/1 -> Switch/1
  Constant1/1 -> Switch1/1

== system FOC1/bldc/Torque Control ==
  f32_TorqueCmd_Nm : Inport
  f32_SpeedAct_rpm : Inport  Port=2
  Kp : Inport  Port=3
  Ki : Inport  Port=4
  TrqMax : Inport  Port=5
  TrqMin : Inport  Port=6
  Enable : EnablePort  StatesWhenEnabling=reset
  Add : Sum  Inputs=+++
  Constant : Constant  Value=0  OutDataTypeStr=single
  Constant1 : Constant  Value=0  OutDataTypeStr=single
  Saturation Dynamic : simulink/Discontinuities/Saturation Dynamic  OutMin=[]  OutMax=[]  OutDataTypeStr=Inherit: Same as second input  OutDataType=fixdt(1, 16)  OutScaling=2^-10  DoSatur=off
  SpdNegLimit : Subsystem
  SpdPosLimit : Subsystem
  Subtract : Sum  Inputs=+-
  Subtract1 : Sum  Inputs=+-
  TrqSet : Outport  OutputWhenDisabled=reset  InitialOutput=0  VectorParamsAs1DForOutWhenUnconnected=off
  wires:
  Saturation Dynamic/1 -> TrqSet/1
  f32_TorqueCmd_Nm/1 -> Add/2, Subtract1/2, Subtract/2
  TrqMax/1 -> Saturation Dynamic/1, Subtract/1
  TrqMin/1 -> Saturation Dynamic/3, Subtract1/1
  Add/1 -> Saturation Dynamic/2
  SpdPosLimit/1(out) -> Add/1
  SpdNegLimit/1(out) -> Add/3
  Kp/1 -> SpdNegLimit/4(Kp), SpdPosLimit/4(Kp)
  Ki/1 -> SpdNegLimit/5(Ki), SpdPosLimit/5(Ki)
  f32_SpeedAct_rpm/1 -> SpdPosLimit/1(f32_SpeedAct_rpm), SpdNegLimit/1(f32_SpeedAct_rpm)
  Constant/1 -> SpdPosLimit/2(max)
  Constant1/1 -> SpdNegLimit/3(min)
  Subtract1/1 -> SpdPosLimit/3(min)
  Subtract/1 -> SpdNegLimit/2(max)

== system FOC1/bldc/FwcFdbCalc/PT1_1 ==
  bin : Inport
  cof : Inport  Port=2
  Constant : Constant  OutDataTypeStr=single
  Product1 : Product  RndMeth=Zero  OutDataTypeStr=Inherit: Same as first input
  Product3 : Product  RndMeth=Zero  OutDataTypeStr=Inherit: Same as first input
  Subtract : Sum  Inputs=-+  OutDataTypeStr=Inherit: Same as first input
  Sum1 : Sum  Inputs=|++  OutDataTypeStr=Inherit: Same as first input
  Unit Delay1 : UnitDelay  SampleTime=-1  HasFrameUpgradeWarning=on
  bout : Outport  VectorParamsAs1DForOutWhenUnconnected=off
  wires:
  Product3/1 -> Sum1/2
  Unit Delay1/1 -> Product3/1
  Product1/1 -> Sum1/1
  bin/1 -> Product1/1
  Constant/1 -> Subtract/2
  cof/1 -> Subtract/1, Product1/2
  Sum1/1 -> bout/1, Unit Delay1/1
  Subtract/1 -> Product3/2

== system FOC1/bldc/PMC_IsDesCalc/FWC ==
  note: 处理优化
  note: 删除限幅
  f32_ModulationReq : Inport
  Ufdb : Inport  Port=2
  Ts : Inport  Port=3
  iDaDesTblLimd : Inport  Port=4
  PMC_iDaDesBs : Inport  Port=5
  PMC_iDaDesMTPV : Inport  Port=6
  Add : Sum  Inputs=-+
  Add1 : Sum  Inputs=-+
  Add2 : Sum
  Chart1 : Stateflow chart  Commented=on  TreatAsAtomicUnit=on
  MATLAB Function1 : MATLAB Function  TreatAsAtomicUnit=on
  Min2 : MinMax  Function=max  Inputs=2
  PI : Subsystem
  Subtract : Sum  Inputs=+-
  Unit Delay1 : UnitDelay  SampleTime=-1  HasFrameUpgradeWarning=on
  PMC_IdDes : Outport  OutputWhenDisabled=reset  InitialOutput=0  VectorParamsAs1DForOutWhenUnconnected=off
  wires:
  PI/1(Kp) -> MATLAB Function1/2(kp)
  Add/1 -> MATLAB Function1/4(MAX)
  Add1/1 -> MATLAB Function1/5(MIN)
  Subtract/1 -> PI/1(error), MATLAB Function1/1(err)
  f32_ModulationReq/1 -> Subtract/1
  Unit Delay1/1 -> MATLAB Function1/6("intg ")
  MATLAB Function1/2(intg) -> Unit Delay1/1
  PI/2(Ki) -> MATLAB Function1/3(ki)
  Ts/1 -> PI/2(Ts)
  PMC_iDaDesBs/1 -> Min2/1
  PMC_iDaDesMTPV/1 -> Add1/2, Min2/2
  Min2/1 -> Add/2
  iDaDesTblLimd/1 -> Add1/1, Add2/2, Add/1
  MATLAB Function1/1(out) -> Add2/1
  Add2/1 -> PMC_IdDes/1
  Ufdb/1 -> Subtract/2

== system FOC1/bldc/PMC_IsDesCalc/MaxI vs Freq ==
  frqElec : Inport
  Abs : Abs  SaturateOnIntegerOverflow=off
  Freq vs MaxI : Lookup_n-D  NumberOfTableDimensions=1  DataSpecification=Lookup table object  LookupTableObject=facIphaMaxFreq_T  BreakpointsForDimension1=[0 1 5 10 20 50 100 200 300 400 800 1600]  BeginIndexSearchUsingPreviousIndexResult=on  Table=[0.5 0.5 0.6 0.7 0.75 0.8 0.85 0.9 0.97 1 1 1]  ExtrapMethod=Clip  UseLastTableValue=on  InternalRulePriority=Speed  OutDataTypeStr=Inherit: Inherit from 'Table data'
  Ismax1 : Constant  Value=g_msgCore0to2_maxCur  OutDataTypeStr=single
  PT1_2 : Subsystem
  Product : Product
  tauPT1IsMax : Constant  Value=0.1  OutDataTypeStr=single
  IsMax : Outport  VectorParamsAs1DForOutWhenUnconnected=off
  wires:
  frqElec/1 -> Abs/1
  PT1_2/1(bout) -> Freq vs MaxI/1
  Ismax1/1 -> Product/1
  Product/1 -> IsMax/1
  tauPT1IsMax/1 -> PT1_2/2(cof)
  Abs/1 -> PT1_2/1(bin)
  Freq vs MaxI/1 -> Product/2

== system FOC1/bldc/PMC_IsDesCalc/PMC_GenSigCalcn ==
  PMC_omSttr : Inport
  Abs : Abs  SaturateOnIntegerOverflow=off
  Divide : Product  Inputs=*/
  MinMax : MinMax  Function=max  Inputs=2
  unit : Constant  OutDataTypeStr=single  SampleTime=-1
  w10Hz : Constant  Value=10*2*pi  OutDataTypeStr=single  SampleTime=-1
  PMC_omSttrRecpr : Outport  SampleTime=Tsw  VectorParamsAs1DForOutWhenUnconnected=off
  wires:
  w10Hz/1 -> MinMax/1
  MinMax/1 -> Divide/2
  Abs/1 -> MinMax/2
  Divide/1 -> PMC_omSttrRecpr/1
  unit/1 -> Divide/1
  PMC_omSttr/1 -> Abs/1

== system FOC1/bldc/PMC_IsDesCalc/PMC_IsdDesCalc ==
  note: 此除参考EP32软件更改
  PMC_psiMax : Inport
  PMC_TrqEmDes : Inport  Port=2
  rotorTemp : Inport  Port=3
  iDaDesTblLimd : Subsystem
  PMC_iDaDesTblLimd : Outport  VectorParamsAs1DForOutWhenUnconnected=off
  PMC_iDaDesBs : Outport  Port=2  VectorParamsAs1DForOutWhenUnconnected=off
  PMC_iDaDesMTPV : Outport  Port=3  VectorParamsAs1DForOutWhenUnconnected=off
  wires:
  iDaDesTblLimd/2(iDaDesTblLimd) -> PMC_iDaDesTblLimd/1
  PMC_TrqEmDes/1 -> iDaDesTblLimd/2(PMC_TrqEmDes)
  PMC_psiMax/1 -> iDaDesTblLimd/1(PMC_psiMax)
  iDaDesTblLimd/3(iDaDesBS) -> PMC_iDaDesBs/1  "BS"
  iDaDesTblLimd/1(iDaDesMTPV) -> PMC_iDaDesMTPV/1  "MTPV"
  rotorTemp/1 -> iDaDesTblLimd/3(rotorTemp)

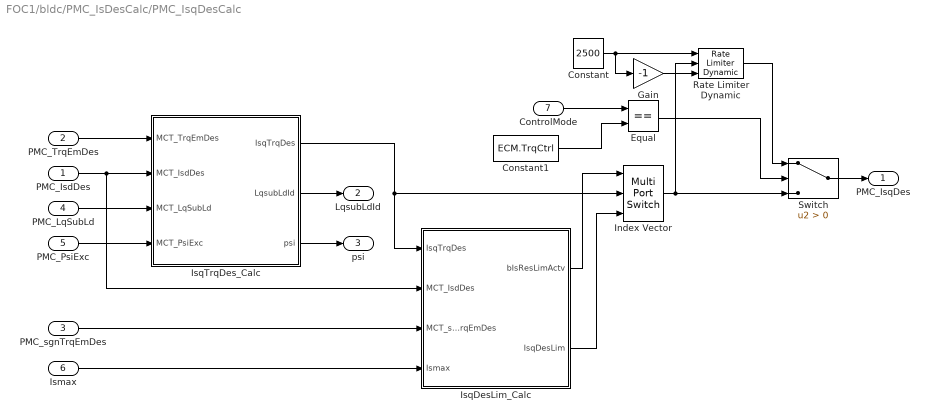
== system FOC1/bldc/PMC_IsDesCalc/PMC_IsqDesCalc ==
  PMC_IsdDes : Inport
  PMC_TrqEmDes : Inport  Port=2
  PMC_sgnTrqEmDes : Inport  Port=3
  PMC_LqSubLd : Inport  Port=4
  PMC_PsiExc : Inport  Port=5
  Ismax : Inport  Port=6
  ControlMode : Inport  Port=7
  Constant : Constant  Value=2500
  Constant1 : Constant  Value=ECM.TrqCtrl
  Equal : RelationalOperator  Operator===  OutDataTypeStr=boolean  RndMeth=Simplest  InputSameDT=off
  Gain : Gain  Gain=-1
  Index Vector : MultiPortSwitch  DataPortOrder=Zero-based contiguous  Inputs=2  zeroidx=on  SaturateOnIntegerOverflow=off  InputSameDT=off
  IsqDesLim_Calc : Subsystem  TreatAsAtomicUnit=on
  IsqTrqDes_Calc : Subsystem  TreatAsAtomicUnit=on
  Rate Limiter Dynamic : simulink/Discontinuities/Rate Limiter Dynamic
  Switch : Switch  Criteria=u2 > Threshold  SaturateOnIntegerOverflow=off  InputSameDT=off
  PMC_IsqDes : Outport  VectorParamsAs1DForOutWhenUnconnected=off
  LqsubLdId : Outport  Port=2
  psi : Outport  Port=3
  wires:
  PMC_sgnTrqEmDes/1 -> IsqDesLim_Calc/3(MCT_sgnTrqEmDes)
  IsqTrqDes_Calc/1(IsqTrqDes) -> IsqDesLim_Calc/1(IsqTrqDes), Index Vector/2
  PMC_IsdDes/1 -> IsqTrqDes_Calc/2(MCT_IsdDes), IsqDesLim_Calc/2(MCT_IsdDes)
  PMC_PsiExc/1 -> IsqTrqDes_Calc/4(MCT_PsiExc)
  PMC_LqSubLd/1 -> IsqTrqDes_Calc/3(MCT_LqSubLd)
  PMC_TrqEmDes/1 -> IsqTrqDes_Calc/1(MCT_TrqEmDes)
  IsqDesLim_Calc/2(IsqDesLim) -> Index Vector/3
  IsqDesLim_Calc/1(bIsResLimActv) -> Index Vector/1
  Ismax/1 -> IsqDesLim_Calc/4(Ismax)
  Index Vector/1 -> Rate Limiter Dynamic/2, Switch/3
  IsqTrqDes_Calc/2(LqsubLdId) -> LqsubLdId/1
  IsqTrqDes_Calc/3(psi) -> psi/1
  Switch/1 -> PMC_IsqDes/1
  Equal/1 -> Switch/2
  Rate Limiter Dynamic/1 -> Switch/1
  Constant/1 -> Gain/1, Rate Limiter Dynamic/1
  Gain/1 -> Rate Limiter Dynamic/3
  ControlMode/1 -> Equal/1
  Constant1/1 -> Equal/2

== system FOC1/bldc/PMC_IsDesCalc/PMC_PwmModCalcn ==
  PMC_uPwmMax : Inport
  PMC_omSttrRecpr : Inport  Port=2
  Product : Product  RndMeth=Zero
  PMC_psiMax : Outport  VectorParamsAs1DForOutWhenUnconnected=off
  wires:
  Product/1 -> PMC_psiMax/1
  PMC_omSttrRecpr/1 -> Product/2
  PMC_uPwmMax/1 -> Product/1

== system FOC1/bldc/PMC_PsmMdl/MCT_GenSigCalcn ==
  ISP_Isd : Inport
  ISP_Isq : Inport  Port=2
  PT1 : MathLib/PT1  SystemSampleTime=-1  VariantActivationTime=update diagram  Latency=0  AutoFrameSizeCalculation=off
  PT2 : MathLib/PT1  SystemSampleTime=-1  VariantActivationTime=update diagram  Latency=0  AutoFrameSizeCalculation=off
  tauPT1Isd : Constant  Value=0.1  OutDataTypeStr=single
  ISP_iDaFild : Outport  VectorParamsAs1DForOutWhenUnconnected=off
  ISP_iQaFild : Outport  Port=2  VectorParamsAs1DForOutWhenUnconnected=off
  wires:
  ISP_Isq/1 -> PT2/1
  PT2/1 -> ISP_iQaFild/1
  tauPT1Isd/1 -> PT2/2, PT1/2
  ISP_Isd/1 -> PT1/1
  PT1/1 -> ISP_iDaFild/1
